simulink model "Tractor_Trailer_SingleTrack_Simulink"  (R2025a)
settings: Solver=VariableStepAuto  StartTime=0.0  StopTime=10.0  RelTol=1e-3
undefined symbols (not defined in the file or in its folder): params
libraries: simulink_extras x1
settings Model: Creator=jakub  LastModifiedBy=jakub
settings SolverCC: AlgebraicLoopSolver=TrustRegion
settings DebuggingCC: UnconnectedInputMsg=warning  UnconnectedOutputMsg=warning  UnconnectedLineMsg=warning
settings ModelReferenceCC: EnableRefExpFcnMdlSchedulingChecks=on
settings RTWCC: GPUComputeCapability=3.5

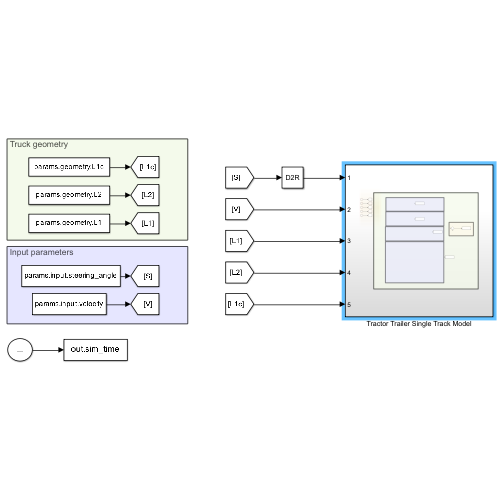
[thumbnail: Simulink's stored preview of the top-level diagram]
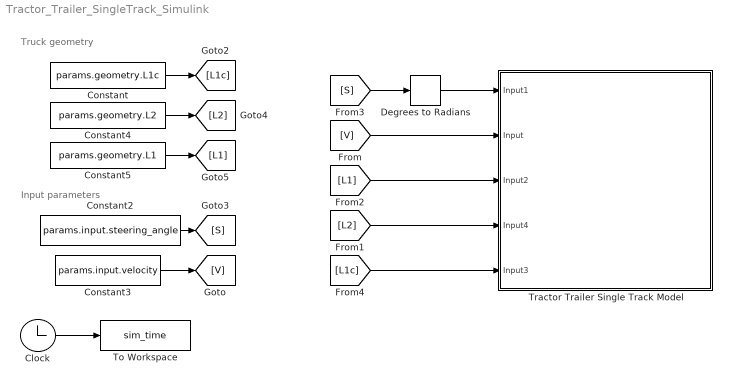
== system Tractor_Trailer_SingleTrack_Simulink ==
  note: Truck geometry
  note: Input parameters
  Clock : Clock
  Constant : Constant  Value=params.geometry.L1c
  Constant2 : Constant  Value=params.input.steering_angle
  Constant3 : Constant  Value=params.input.velocity
  Constant4 : Constant  Value=params.geometry.L2
  Constant5 : Constant  Value=params.geometry.L1
  Degrees to Radians : simulink_extras/Transformations/Degrees to Radians
  To Workspace : ToWorkspace  VariableName=sim_time  SaveFormat=Timeseries  SampleTime=-1
  Tractor Trailer Single Track Model : Subsystem
  wires:
  Clock/1 -> To Workspace/1
  Constant/1 -> [L1c]
  Constant2/1 -> [S]
  Constant3/1 -> [V]
  [V] -> Tractor Trailer Single Track Model/2(Input)
  Constant4/1 -> [L2]
  Constant5/1 -> [L1]
  [L1c] -> Tractor Trailer Single Track Model/5(Input3)
  [S] -> Degrees to Radians/1
  Degrees to Radians/1 -> Tractor Trailer Single Track Model/1(Input1)
  [L1] -> Tractor Trailer Single Track Model/3(Input2)
  [L2] -> Tractor Trailer Single Track Model/4(Input4)

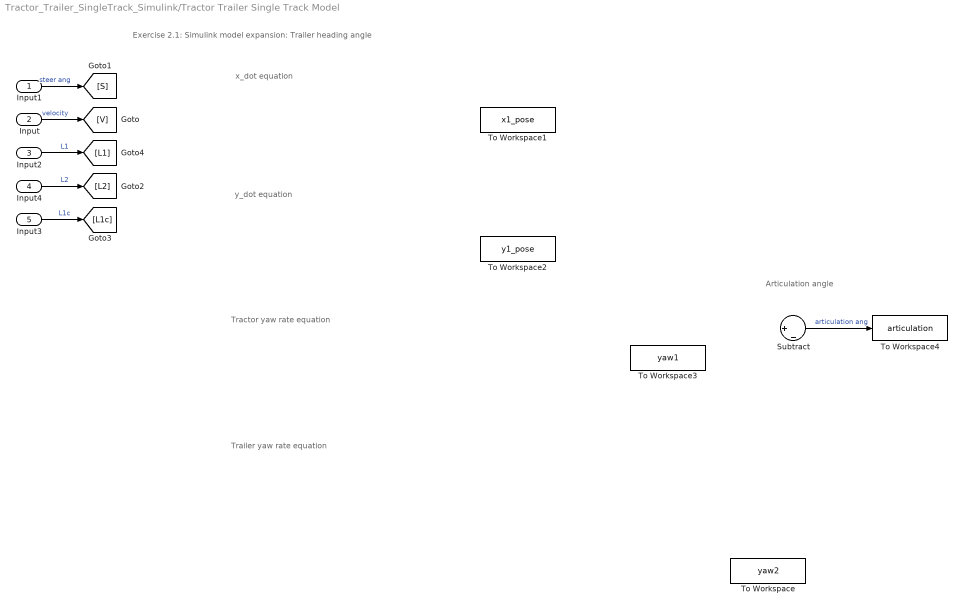
== system Tractor_Trailer_SingleTrack_Simulink/Tractor Trailer Single Track Model ==
  note: Exercise 2.1: Simulink model expansion: Trailer heading angle
  note: Articulation angle
  note: y_dot equation
  note: x_dot equation
  note: Tractor yaw rate equation
  note: Trailer yaw rate equation
  Input1 : Inport
  Input : Inport  Port=2
  Input2 : Inport  Port=3
  Input4 : Inport  Port=4
  Input3 : Inport  Port=5
  Subtract : Sum  Inputs=||+|-
  To Workspace : ToWorkspace  VariableName=yaw2  SaveFormat=Timeseries  SampleTime=-1
  To Workspace1 : ToWorkspace  VariableName=x1_pose  SaveFormat=Timeseries  SampleTime=-1
  To Workspace2 : ToWorkspace  VariableName=y1_pose  SaveFormat=Timeseries  SampleTime=-1
  To Workspace3 : ToWorkspace  VariableName=yaw1  SaveFormat=Timeseries  SampleTime=-1
  To Workspace4 : ToWorkspace  VariableName=articulation  SaveFormat=Timeseries  SampleTime=-1
  wires:
  Input/1 -> [V]  "velocity"
  Input1/1 -> [S]  "steer ang"
  Input2/1 -> [L1]  "L1"
  Subtract/1 -> To Workspace4/1  "articulation ang"
  Input4/1 -> [L2]  "L2"
  Input3/1 -> [L1c]  "L1c"
